simulink model "sim_bandpass_singleBand"  (R2024b)
settings: Solver=FixedStepDiscrete  StartTime=0.0  StopTime=inf  RelTol=1e-3  EnableMultiTasking=on
values from neighbouring files (symbols this model uses):
  sm =     [reference_output.mat]
undefined symbols (not defined in the file or in its folder): fdesignblkfcn, gcbh
settings Model: Creator=ronens  LastModifiedBy=hardeep
settings SolverCC: AlgebraicLoopSolver=TrustRegion
settings DataIOCC: LimitDataPoints=on  SaveFormat=Array  SignalLoggingSaveFormat=ModelDataLogs  ReturnWorkspaceOutputs=off
settings OptimizationCC: ExpressionDepthLimit=2147483647  LifeSpan=inf
settings DebuggingCC: UnderspecifiedInitializationDetection=Classic  MergeDetectMultiDrivingBlocksExec=none  SolverPrmCheckMsg=warning  ParameterPrecisionLossMsg=none  FcnCallInpInsideContextMsg=warning  UnconnectedInputMsg=warning  UnconnectedOutputMsg=warning  UnconnectedLineMsg=warning  StateNameClashWarn=warning  SFUnexpectedBacktrackingDiag=warning  SFNoUnconditionalDefaultTransitionDiag=warning  SFExecutionAtInitializationDiag=none  ArithmeticOperatorsInVariantConditions=warning
settings HardwareCC: ProdBitPerPointer=32  ProdBitPerSizeT=32  ProdBitPerPtrDiffT=32  ProdLargestAtomicFloat=None  ProdIntDivRoundTo=Undefined  ProdEndianess=Unspecified  ProdWordSize=32  ProdHWDeviceType=32-bit Generic
settings ModelReferenceCC: EnableRefExpFcnMdlSchedulingChecks=on  PropagateSignalLabelsOutOfModel=off
settings SFSimCC: SimUseLocalCustomCode=off  CustomCodeUndefinedFunction=UseInterfaceOnly
settings RTWCC: RTWUseLocalCustomCode=off  GPUComputeCapability=3.5
settings CodeAppCC: StateflowObjectComments=on
settings GRTTargetCC: TargetLangStandard=C89/C90 (ANSI)
settings ConfigComp: CovMetricSettings=dw  CovSaveCumulativeToWorkspaceVar=on  CovSaveSingleToWorkspaceVar=on  CovExternalEMLEnable=off
settings SimscapeCC: SimscapeNormalizeSystem=off
settings ConfigurationSet: Description=SimMechanics 2G

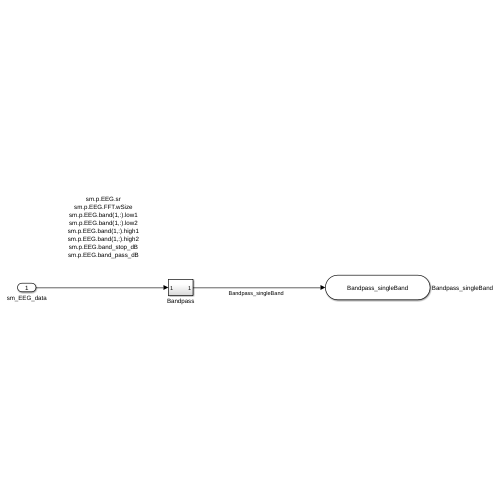
[thumbnail: Simulink's stored preview of the top-level diagram]
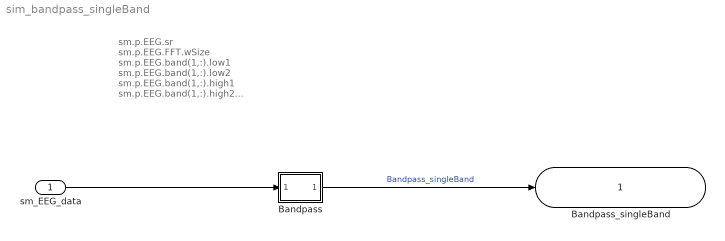
== system sim_bandpass_singleBand ==
  note: sm.p.EEG.sr
      | sm.p.EEG.FFT.wSize
      | sm.p.EEG.band(1,:).low1
      | sm.p.EEG.band(1,:).low2
      | sm.p.EEG.band(1,:).high1
      | sm.p.EEG.band(1,:).high2
      | sm.p.EEG.band_stop_dB
      | sm.p.EEG.band_pass_dB
  sm_EEG_data : Inport  SampleTime=1/sm.p.EEG.sr
  Bandpass : Subsystem
  Bandpass_singleBand : Outport  SignalName=Bandpass_singleBand
  wires:
  sm_EEG_data/1 -> Bandpass/1(In1)
  Bandpass/1(Out1) -> Bandpass_singleBand/1  "Bandpass_singleBand"

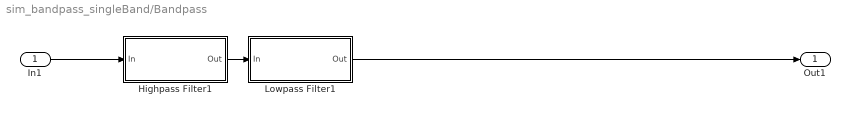
== system sim_bandpass_singleBand/Bandpass ==
  In1 : Inport
  Highpass Filter1 : Subsystem  DialogController=fdesignblkfcn  InitFcn=fdesignblkfcn(gcbh, {'InitFcn'});  mask(Highpass Filter){}
      mask help: Design a highpass filter
      settings: CopyFcn=fdesignblkfcn(gcbh, {'CopyFcn'});
      mask Help: helpview(mapfilelocation('dsp'), 'dsphighpassfilter');
      mask Display: disp('Highpass')
  Lowpass Filter1 : Subsystem  DialogController=fdesignblkfcn  InitFcn=fdesignblkfcn(gcbh, {'InitFcn'});  mask(Lowpass Filter){}
      mask help: Design a lowpass filter
      settings: CopyFcn=fdesignblkfcn(gcbh, {'CopyFcn'});
      mask Help: helpview(mapfilelocation('dsp'), 'dsplowpassfilter');
      mask Display: disp('Lowpass')
  Out1 : Outport
  wires:
  In1/1 -> Highpass Filter1/1(In)
  Highpass Filter1/1(Out) -> Lowpass Filter1/1(In)
  Lowpass Filter1/1(Out) -> Out1/1

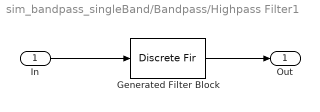
== system sim_bandpass_singleBand/Bandpass/Highpass Filter1 ==
  In : Inport
  Generated Filter Block : DiscreteFir  Tag=BlockMethodSubSystem  Coefficients=[-0.00205792891744371528 0.0153154222464366475 -0.00960983741400391576 -0.00725590434265008244 -0.00266163531845228524 0.00063307152579651616 0.00239923116968173301 0.00292200930180396565 0.00257813667718700696 0.00171958936877448414 0.000657619373084450507 -0.00036230184552082592 -0.00116217812573669735 -0.00163730385542034448 -0.00174608926134487796 -0.00151761145291934578 -0.00102044158499516925 -0.000363899764133448296 0.00033322636753844282 0.000944857807243449071 0.00137111720219415664 0.00153578699605095496 0.00141843189931842284 0.00103826935516446303 0.000466106809154684756 -0.000202557058637173288 -0.000841525618238256031 -0.00133750677285483007 -0.00159201701384797576 -0.0015570529196145494 -0.00122537200132960501 -0.000655674636739894397 5.81101402583800083e-05 0.000782246996928758517 0.00138741698600648115 0.00174989025566010857 0.00179724909444732225 0.00150115579528990219 0.000909795590805156018 0.000117496136143777893 -0.000727433800359344866 -0.00147259957511691394 -0.00196379919088204629 -0.00210377031161549386 -0.00184477444174241845 -0.00122526450552477373 -0.00033913816805900476 0.000647063005878013484 0.00155748598805688951 0.0022072712564416945 0.00246777205827023892 0.00226073789662370721 0.00161638300197598415 0.00062826176471244275 -0.000520832971052246794 -0.0016289672593404541 -0.00246812513701046097 -0.00288172144235434051 -0.00275525357100913325 -0.00210181456468885733 -0.00100504396525064412 0.000323150906217507415 0.00167002640597557501 0.00273869686028643681 0.00335506569839225197 0.00334112714249767181 0.00269055966151931321 0.00150887771697866594 -5.4466340188507528e-05 -0.00164005509787616319 -0.00302104385082982169 -0.00388873878490949296 -0.00403441316907136166 -0.00342688938290929305 -0.00214252650060339604 -0.000361133649233552525 0.0015707018488946259 0.00329172987004931403 0.00447466864168817591 0.00487624285033256936 0.0043510896374754594 0.00295688468306684864 0.000925944759197539304 -0.00138002336410327029 -0.00355422788070166055 -0.0051719047426842385 -0.00588721712977384286 -0.0055026674663301153 -0.00404005917912624371 -0.00172194883255040367 0.00105567997492862645 0.00380020126977283126 0.00598392100189315893 0.00715206892606114371 0.0070103910386935071 0.00550852514196317235 0.00285064130932942677 -0.000523443956139861576 -0.00402087594928168292 -0.00698522659272953709 -0.00881568300264949124 -0.00907342398198066231 -0.00759276649912361563 -0.00452956755468412846 -0.000356808804781541717 0.00421414005414491068 0.00834079758724234205 0.0111983894471403677 0.0121280357712165408 0.0107815534877395529 0.00720700603677587072 0.00187597043389246191 -0.00436719314872661621 -0.010414809171156671 -0.015081669893945061 -0.0173171971934780802 -0.016406275067896943 -0.0121234329969982808 -0.00483776476996090801 0.00448263702781598328 0.0143731790359319152 0.0230512731512883089 0.028651297101641042 0.0295117112682215833 0.0244560716467733114 0.0129930367659959189 -0.00454725405073080641 -0.0269878989889643858 -0.0524091662621303592 -0.0783985198839300956 -0.102272203073153392 -0.121499277198842681 -0.133966163096269908 0.861720752467901918 -0.133966163096269908 -0.121499277198842681 -0.102272203073153392 -0.0783985198839300956 -0.0524091662621303592 -0.0269878989889643858 -0.00454725405073080641 0.0129930367659959189 0.0244560716467733114 0.0295117112682215833 0.028651297101641042 0.0230512731512883089 0.0143731790359319152 0.00448263702781598328 -0.00483776476996090801 -0.0121234329969982808 -0.016406275067896943 -0.0173171971934780802 -0.015081669893945061 -0.010414809171156671 -0.00436719314872661621 0.00187597043389246191 0.00720700603677587072 0.0107815534877395529 0.0121280357712165408 0.0111983894471403677 0.00834079758724234205 0.00421414005414491068 -0.000356808804781541717 -0.00452956755468412846 -0.00759276649912361563 -0.00907342398198066231 -0.00881568300264949124 -0.00698522659272953709 -0.00402087594928168292 -0.000523443956139861576 0.00285064130932942677 ...(+2263 chars)]  InputProcessing=Columns as channels (frame based)
  Out : Outport
  wires:
  Generated Filter Block/1 -> Out/1
  In/1 -> Generated Filter Block/1

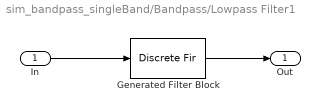
== system sim_bandpass_singleBand/Bandpass/Lowpass Filter1 ==
  In : Inport
  Generated Filter Block : DiscreteFir  Tag=BlockMethodSubSystem  Coefficients=[-0.0010380426683483596 -0.00146443808367044425 -0.00219609942313726521 -0.00286141608919620802 -0.00328868358303058012 -0.00331722410709538824 -0.00284235534322986724 -0.0018525074316127169 -0.000450057313437833215 0.00115666669149118331 0.00269100352499518185 0.00386962854514945071 0.00446903449655085706 0.00438566723588878701 0.0036694668647830179 0.00251819659186405722 0.00122981922980183191 0.000133186221484622806 -0.000502530923492172221 -0.000539284575155045886 -5.8975538171443045e-06 0.000904536369670852253 0.00189433071075950036 0.0026422417911439876 0.00290173585738880569 0.00257243180632245761 0.0017345040323154435 0.000626278588918342339 -0.000424883570781014227 -0.00110300590195973585 -0.00120032446569823498 -0.000686060666070932297 0.000279418467930887154 0.00138929515056794507 0.00228263716376794724 0.00265549931774851627 0.0023610661495839136 0.00145986687070855689 0.00020986283713508638 -0.0010096892044135098 -0.00181399367871689981 -0.00193574247638442069 -0.0013158188966415304 -0.000130095706498169179 0.00125664075961435954 0.0023998869952043078 0.00291473693401803589 0.00260226901989199337 0.00152131716561466532 -1.85631049291437548e-05 -0.00154571746832446845 -0.0025711373070085781 -0.00274492409528188886 -0.00197570376804977752 -0.000471936997594364811 0.0013115069129430168 0.00280811818147334597 0.0035179028703769908 0.00317101086960749944 0.00182651110524243722 -0.000131342409229173854 -0.00210146309841865433 -0.00344943512774456519 -0.00371081486793702628 -0.00274953626730857275 -0.00081802213394766227 0.00150519700811635807 0.00348590540195197873 0.00446391395907901663 0.00406998822943579683 0.00236012808431297237 -0.000180789611935583281 -0.00277377540884432951 -0.00458210647476904685 -0.00497907802453976395 -0.00376174755851296999 -0.00123887658266973199 0.00184088835845239119 0.00450776516823947915 0.00587201080731752055 0.00541651551409107288 0.00318479428873802298 -0.000200985052163455834 -0.00370835230551213885 -0.00620458374264313238 -0.00681758013851369721 -0.00523356379675880487 -0.00183260354296480585 0.00239163439880910695 0.0061151405755530807 0.00809104092761136692 0.00755797475019218731 0.00451892835081623388 -0.000208670830250798687 -0.00520114243387191557 -0.00884674720083710765 -0.00985348441381976407 -0.00769043047427980103 -0.00281681100020991218 0.00338987212197046275 0.00900580942702875441 0.0121374404806233356 0.0115350839442471716 0.00705196355754116305 -0.00020943883747561793 -0.00813578251489699075 -0.0141844156331577091 -0.0161561585502138852 -0.0129349678588911148 -0.0049626244529689667 0.00572430480980518248 0.0159493030057087058 0.0222540738973561469 0.0219443171834096534 0.0140324810394420602 -0.000207243408775494486 -0.0172697575438250026 -0.0320835307314315948 -0.039182536340341842 -0.0341108465702660846 -0.0147017080564396264 0.0181154742734965096 0.060222110669666859 0.104997268104532707 0.144652302252226694 0.171907770496167067 0.18161233114834896 0.171907770496167067 0.144652302252226694 0.104997268104532707 0.060222110669666859 0.0181154742734965096 -0.0147017080564396264 -0.0341108465702660846 -0.039182536340341842 -0.0320835307314315948 -0.0172697575438250026 -0.000207243408775494486 0.0140324810394420602 0.0219443171834096534 0.0222540738973561469 0.0159493030057087058 0.00572430480980518248 -0.0049626244529689667 -0.0129349678588911148 -0.0161561585502138852 -0.0141844156331577091 -0.00813578251489699075 -0.00020943883747561793 0.00705196355754116305 0.0115350839442471716 0.0121374404806233356 0.00900580942702875441 0.00338987212197046275 -0.00281681100020991218 -0.00769043047427980103 -0.00985348441381976407 -0.00884674720083710765 -0.00520114243387191557 -0.000208670830250798687 0.00451892835081623388 0.00755797475019218731 0.00809104092761136692 0.0061151405755530807 0.00239163439880910695 -0.00183260354296480585 -0.00523356379675880487 -0.00681758013851369721 -0.00620458374264313238 -0.00370835230551213885 -0.000200985052163455834 0.00318479428873802298 ...(+1904 chars)]  InputProcessing=Columns as channels (frame based)
  Out : Outport
  wires:
  In/1 -> Generated Filter Block/1
  Generated Filter Block/1 -> Out/1
